simulink subsystem "HEVP2SSC"  (R2025b)
settings: Solver=VariableStepAuto  StartTime=0.0  StopTime=10.0  RelTol=1e-3
undefined symbols (not defined in the file): PlntCltch1Prs, PlntCltch1TimeCnst, PlntCltch1VelTol
libraries: fl_lib x6, nesl_utility_internal x3, simulink x2, sdl_lib x1
settings Model: ModifiedByFormat=The MathWorks, Inc.  Creator=The MathWorks, Inc.  LastModifiedBy=The MathWorks, Inc.
settings OptimizationCC: ReuseModelBlockBuffer=off
settings RTWCC: GPUComputeCapability=3.5

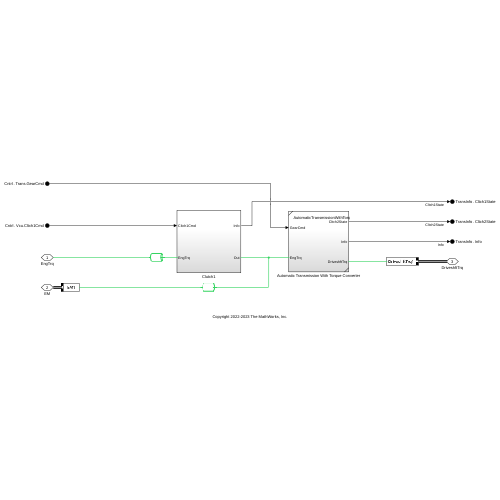
[thumbnail: Simulink's stored preview of the top-level diagram]
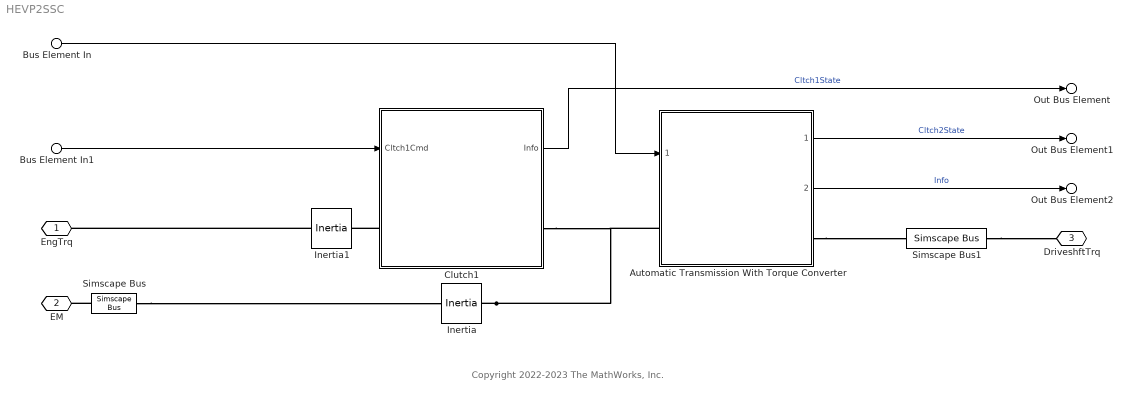
== system HEVP2SSC ==
  note: Copyright 2022-2023 The MathWorks, Inc.
  Bus Element In : Inport  PortName=Cntrl  Element=Trans.GearCmd
  Bus Element In1 : Inport  PortName=Cntrl  Element=Vcu.Cltch1Cmd
  Automatic Transmission With Torque Converter : Subsystem  ReferencedSubsystem=AutomaticTransmissionWithTorqueConverterSSC
  Clutch1 : Subsystem
  Inertia : fl_lib/Mechanical/Rotational Elements/Inertia  inertia=PlntEM1RotInertia kg*m^2  num_ports=foundation.enum.numPorts2.two  w_specify=off  w_priority=High  w=0 rad/s  w_nominal_specify=off  w_nominal_value=1  w_nominal_unit=rad/s  t_specify=off  t_priority=None  t=0 N*m  t_nominal_specify=off  t_nominal_value=1  t_nominal_unit=N*m
      settings: InternalSimscapePortConfiguration="{\"Bottom\":[],\"Left\":[{\"id\":\"I\",\"label\":\"\",\"type\":\"foundation.mechanical.rotational.rotational\"}],\"Right\":[{\"id\":\"J\",\"label\":\"\",\"type\":\"foundation.mechanical.rotational.rotational\"}],\"Top\":[]}"
  Inertia1 : fl_lib/Mechanical/Rotational Elements/Inertia  inertia=PlntEngInertia kg*m^2  num_ports=foundation.enum.numPorts2.two  w_specify=off  w_priority=High  w=0 rad/s  w_nominal_specify=off  w_nominal_value=1  w_nominal_unit=rad/s  t_specify=off  t_priority=None  t=0 N*m  t_nominal_specify=off  t_nominal_value=1  t_nominal_unit=N*m
      settings: InternalSimscapePortConfiguration="{\"Bottom\":[],\"Left\":[{\"id\":\"I\",\"label\":\"\",\"type\":\"foundation.mechanical.rotational.rotational\"}],\"Right\":[{\"id\":\"J\",\"label\":\"\",\"type\":\"foundation.mechanical.rotational.rotational\"}],\"Top\":[]}"
  Simscape Bus : SimscapeBus  HierarchyStrings=EM1
  Simscape Bus1 : SimscapeBus  HierarchyStrings=DriveshftTrq1
  EngTrq : PMIOPort  Side=Left
  EM : PMIOPort  Port=2  Side=Left
  DriveshftTrq : PMIOPort  Port=3  Side=Right
  Out Bus Element : Outport  PortName=TransInfo  Element=Cltch1State
  Out Bus Element1 : Outport  PortName=TransInfo  Element=Cltch2State
  Out Bus Element2 : Outport  PortName=TransInfo  Element=Info
  wires:
  Clutch1/1(Info) -> Out Bus Element/1  "Cltch1State"
  Bus Element In/1 -> Automatic Transmission With Torque Converter/1
  Automatic Transmission With Torque Converter/2 -> Out Bus Element2/1  "Info"
  Automatic Transmission With Torque Converter/1 -> Out Bus Element1/1  "Cltch2State"
  Bus Element In1/1 -> Clutch1/1(Cltch1Cmd)
  connections:
  Inertia/LConn1 -- Automatic Transmission With Torque Converter/LConn1 -- Clutch1/RConn1
  Inertia1/RConn1 -- EngTrq/RConn1
  Simscape Bus/LConn1 -- Inertia/RConn1
  Simscape Bus/RConn1 -- EM/RConn1
  Simscape Bus1/RConn1 -- DriveshftTrq/RConn1
  Clutch1/LConn1 -- Inertia1/LConn1
  Automatic Transmission With Torque Converter/RConn1 -- Simscape Bus1/LConn1

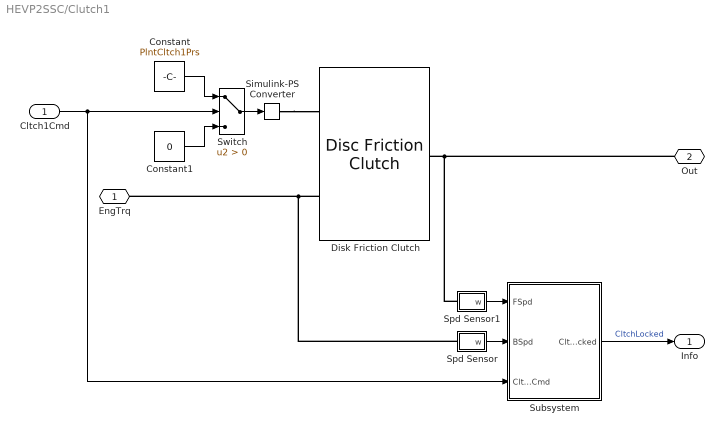
== system HEVP2SSC/Clutch1 ==
  Cltch1Cmd : Inport
  Constant : Constant  Value=PlntCltch1Prs  SampleTime=-1
  Constant1 : Constant  Value=0  SampleTime=-1
  Disk Friction Clutch : sdl_lib/Clutches/Disc Friction Clutch  geometry_model=sdl.enum.friction_geometry.radius  r_eff=PlntCltch1Radius m  d_o=150 mm  d_i=100 mm  nS=PlntCltch1NumDisk  piston_area=PlntCltch1AppPrsArea m^2  unidirectional=sdl.enum.directionality.bidirectional  friction_model=sdl.enum.friction_model_TLU_thermal.fixed  mu_w_vector=[0, 100, 1000] rad/s  temperature_TLU=[280, 300, 320] K  mu_static=PlntCltch1StatFric  mu_static_vector=[.4, .38, .36]  mu_coulomb=PlntCltch1KinFric  mu_coulomb_vector=[.3, .22, .19]  mu_coulomb_temp_vector=[.3, .28, .25]  mu_coulomb_matrix=[.34, .32, .3; .3, .28, .25; .25, .2, .15]  mu_interp_method=simscape.enum.interpolation.linear  mu_extrap_method=simscape.enum.extrapolation.linear  d_f=PlntCltch1DerateFctr  w_tol=PlntCltch1VelTol rad/s  pressure_min=PlntCltch1EngdPrs Pa  mu_visc=PlntCltch1InDamp N*m*s/rad  initial_state_locked=sdl.enum.initial_lock.unlocked  thermal_mass=50 kJ/K  T_init=300 K
      settings: InternalSimscapePortConfiguration="{\"Bottom\":[],\"Left\":[{\"id\":\"P\",\"label\":\"P\",\"type\":\"input\"},{\"id\":\"B\",\"label\":\"B\",\"type\":\"foundation.mechanical.rotational.rotational\"}],\"Right\":[{\"id\":\"F\",\"label\":\"F\",\"type\":\"foundation.mechanical.rotational.rotational\"}],\"Top\":[]}"
  Simulink-PS Converter : nesl_utility_internal/Simulink-PS Converter  PhysicalDomain=network_engine_domain  SubClassName=ps_input  LeftPortType=input  RightPortType=output  PseudoPeriodic=off  Frequencies=[]  NoiseDistribution=none  NoiseParameters=[]  Unit=Pa  AffineConversion=off  FilteringAndDerivatives=filter  SimscapeFilterOrder=1  InputFilterTimeConstant=PlntCltch1TimeCnst*3  UdotUserProvided=0
  Spd Sensor : Subsystem
  Spd Sensor1 : Subsystem
  Subsystem : Subsystem
  Switch : Switch  Criteria=u2 > Threshold  ZeroCross=off  SaturateOnIntegerOverflow=off  InputSameDT=off
  EngTrq : PMIOPort  Side=Left
  Out : PMIOPort  Port=2  Side=Right
  Info : Outport  VectorParamsAs1DForOutWhenUnconnected=off
  wires:
  Constant/1 -> Switch/1
  Constant1/1 -> Switch/3
  Switch/1 -> Simulink-PS Converter/1
  Spd Sensor1/1(w) -> Subsystem/1(FSpd)
  Subsystem/1(CltchLocked) -> Info/1  "CltchLocked"
  Cltch1Cmd/1 -> Subsystem/3(CltchCmd), Switch/2
  Spd Sensor/1(w) -> Subsystem/2(BSpd)
  connections:
  Disk Friction Clutch/LConn2 -- Spd Sensor/LConn1 -- EngTrq/RConn1
  Out/RConn1 -- Spd Sensor1/LConn1 -- Disk Friction Clutch/RConn1
  Simulink-PS Converter/RConn1 -- Disk Friction Clutch/LConn1

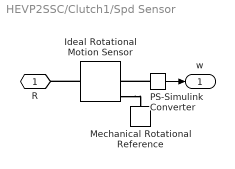
== system HEVP2SSC/Clutch1/Spd Sensor ==
  Ideal Rotational Motion Sensor : fl_lib/Mechanical/Mechanical Sensors/Ideal Rotational Motion Sensor  reference=foundation.enum.MeasurementReference.difference  acceleration_port=false  velocity_port=true  position_port=true  wrap_angle=simscape.enum.onoff.off  offset=0 rad
  Mechanical Rotational Reference : fl_lib/Mechanical/Rotational Elements/Mechanical Rotational Reference
  PS-Simulink Converter : nesl_utility_internal/PS-Simulink Converter  PhysicalDomain=network_engine_domain  SubClassName=ps_output  LeftPortType=input  RightPortType=output  PseudoPeriodic=off  Frequencies=[]  VectorFormat=inherit  Unit=inherit  AffineConversion=off
  R : PMIOPort  Side=Left
  w : Outport
  wires:
  PS-Simulink Converter/1 -> w/1
  connections:
  Ideal Rotational Motion Sensor/RConn1 -- Mechanical Rotational Reference/LConn1
  Ideal Rotational Motion Sensor/LConn1 -- R/RConn1
  PS-Simulink Converter/LConn1 -- Ideal Rotational Motion Sensor/RConn2

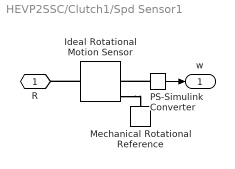
== system HEVP2SSC/Clutch1/Spd Sensor1 ==
  Ideal Rotational Motion Sensor : fl_lib/Mechanical/Mechanical Sensors/Ideal Rotational Motion Sensor  reference=foundation.enum.MeasurementReference.difference  acceleration_port=false  velocity_port=true  position_port=true  wrap_angle=simscape.enum.onoff.off  offset=0 rad
  Mechanical Rotational Reference : fl_lib/Mechanical/Rotational Elements/Mechanical Rotational Reference
  PS-Simulink Converter : nesl_utility_internal/PS-Simulink Converter  PhysicalDomain=network_engine_domain  SubClassName=ps_output  LeftPortType=input  RightPortType=output  PseudoPeriodic=off  Frequencies=[]  VectorFormat=inherit  Unit=inherit  AffineConversion=off
  R : PMIOPort  Side=Left
  w : Outport
  wires:
  PS-Simulink Converter/1 -> w/1
  connections:
  Ideal Rotational Motion Sensor/RConn1 -- Mechanical Rotational Reference/LConn1
  Ideal Rotational Motion Sensor/LConn1 -- R/RConn1
  PS-Simulink Converter/LConn1 -- Ideal Rotational Motion Sensor/RConn2

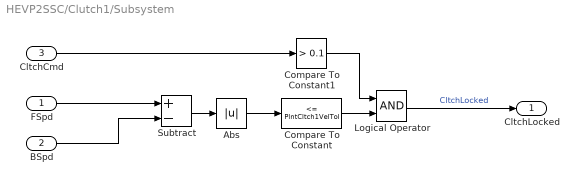
== system HEVP2SSC/Clutch1/Subsystem ==
  FSpd : Inport
  BSpd : Inport  Port=2
  CltchCmd : Inport  Port=3
  Abs : Abs  ZeroCross=off  SaturateOnIntegerOverflow=off
  Compare To Constant : simulink/Logic and Bit Operations/Compare To Constant  relop=<=  const=PlntCltch1VelTol  OutDataTypeStr=boolean  ZeroCross=off
  Compare To Constant1 : simulink/Logic and Bit Operations/Compare To Constant  relop=>  const=0.1  OutDataTypeStr=boolean  ZeroCross=off
  Logical Operator : Logic  AllPortsSameDT=off  OutDataTypeStr=boolean
  Subtract : Sum  Inputs=+-
  CltchLocked : Outport
  wires:
  Logical Operator/1 -> CltchLocked/1  "CltchLocked"
  Compare To Constant/1 -> Logical Operator/2
  CltchCmd/1 -> Compare To Constant1/1
  Subtract/1 -> Abs/1
  Abs/1 -> Compare To Constant/1
  Compare To Constant1/1 -> Logical Operator/1
  FSpd/1 -> Subtract/1
  BSpd/1 -> Subtract/2
